simulink model "UUV_PID_Control_Model"  (R2019b)
settings: Solver=VariableStepAuto  StartTime=0.0  StopTime=12  RelTol=1e-3
undefined symbols (not defined in the file): dr, drr, dx, dxx, dz, dzz, g, kdr, kds, kdx, kdz, kf, kir, kis, kix, kiz, kpr, kps, kpx, kpz, L, mr, mx, mz, r, Ud, waypoints
libraries: simulink x2
settings Model: Creator=7385281  LastModifiedBy=7385281
settings SolverCC: ZeroCrossAlgorithm=Adaptive
settings DataIOCC: ReturnWorkspaceOutputs=off
settings DebuggingCC: IgnoredZcDiagnostic=none

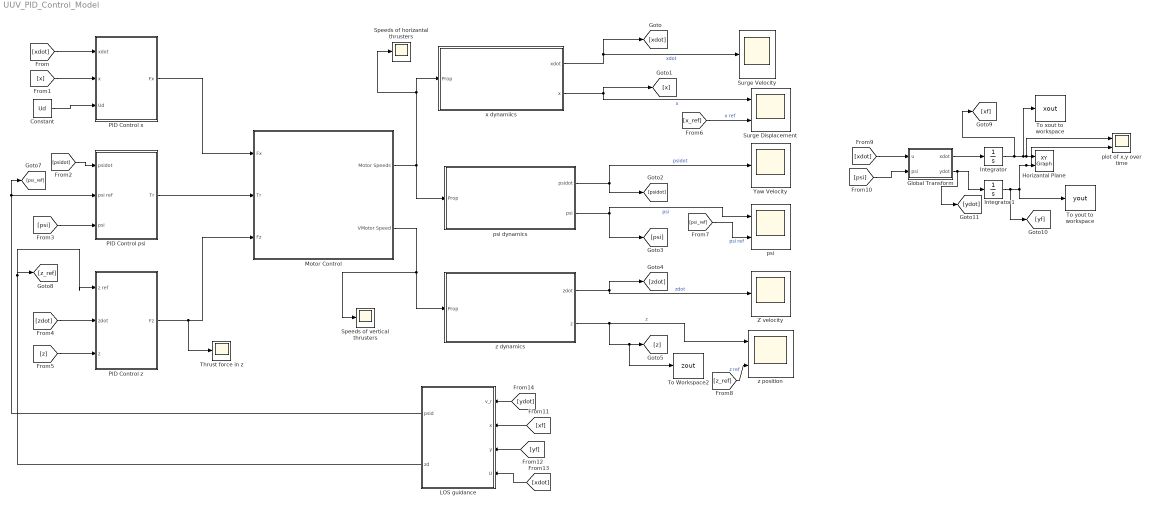
== system UUV_PID_Control_Model ==
  Constant : Constant  Value=Ud
  Global Transform : MATLAB Function  TreatAsAtomicUnit=on
  Horizantal Plane : simulink/Sinks/XY Graph  xmin=-5  xmax=5  ymin=-5  ymax=5  st=-1
  Integrator : Integrator
  Integrator1 : Integrator
  LOS guidance : Subsystem
  Motor Control : Subsystem
  PID Control psi : Subsystem
  PID Control x : Subsystem
  PID Control z : Subsystem
  Speeds of horizantal thrusters : Scope
  Speeds of vertical thrusters : Scope
  Surge Displacement : Scope  NumInputPorts=2
  Surge Velocity : Scope
  Thrust force in z : Scope
  To Workspace2 : ToWorkspace  VariableName=zout  SampleTime=-1
      settings: Save2DSignal=2-D array (concatenate along first dimension)
  To xout to workspace : ToWorkspace  VariableName=xout  SampleTime=-1
      settings: Save2DSignal=2-D array (concatenate along first dimension)
  To yout to workspace : ToWorkspace  VariableName=yout  SampleTime=-1
      settings: Save2DSignal=2-D array (concatenate along first dimension)
  Yaw Velocity : Scope
  Z velocity : Scope
  plot of x,y over time : Scope  NumInputPorts=2
  psi : Scope  NumInputPorts=2
  psi dynamics : Subsystem
  x dynamiics : Subsystem
  z dynamics : Subsystem
  z position : Scope  NumInputPorts=2
  wires:
  x dynamiics/1(xdot) -> [xdot], Surge Velocity/1  "xdot"
  x dynamiics/2(x) -> Surge Displacement/1, [x]  "x"
  psi dynamics/2(psi) -> [psi], psi/1  "psi"
  psi dynamics/1(psidot) -> Yaw Velocity/1, [psidot]  "psidot"
  z dynamics/1(zdot) -> [zdot], Z velocity/1  "zdot"
  z dynamics/2(z) -> z position/1, To Workspace2/1, [z]  "z"
  Motor Control/2(VMotor Speed) -> Speeds of vertical thrusters/1, z dynamics/1(Prop)
  PID Control x/1(Fx) -> Motor Control/1(Fx)
  LOS guidance/1(psid) -> [psi_ref], PID Control psi/2(psi ref)
  PID Control psi/1(Tr) -> Motor Control/2(Tr)
  LOS guidance/2(zd) -> PID Control z/1(z ref), [z_ref]
  PID Control z/1(Fz) -> Thrust force in z/1, Motor Control/3(Fz)
  [xdot] -> PID Control x/1(xdot)
  [x] -> PID Control x/2(x)
  [psidot] -> PID Control psi/1(psidot)
  [psi] -> PID Control psi/3(psi)
  [zdot] -> PID Control z/2(zdot)
  [z] -> PID Control z/3(z)
  [x_ref] -> Surge Displacement/2  "x ref"
  [psi_ref] -> psi/2  "psi ref"
  [z_ref] -> z position/2  "z ref"
  Global Transform/1(xdot) -> Integrator/1
  Global Transform/2(ydot) -> [ydot], Integrator1/1
  [xdot] -> Global Transform/1(u)
  [psi] -> Global Transform/2(psi)
  Integrator/1 -> [xf], To xout to workspace/1, plot of x,y over time/1, Horizantal Plane/1
  Integrator1/1 -> [yf], plot of x,y over time/2, Horizantal Plane/2, To yout to workspace/1
  [xf] -> LOS guidance/2(x)
  [yf] -> LOS guidance/3(y)
  [xdot] -> LOS guidance/4(U)
  [ydot] -> LOS guidance/1(v_r)
  Constant/1 -> PID Control x/3(Ud)
  Motor Control/1(Motor Speeds) -> Speeds of horizantal thrusters/1, x dynamiics/1(Prop), psi dynamics/1(Prop)

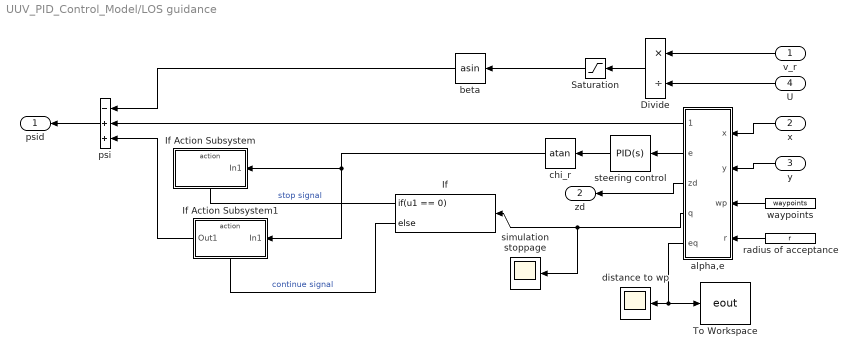
== system UUV_PID_Control_Model/LOS guidance ==
  v_r : Inport
  x : Inport  Port=2
  y : Inport  Port=3
  U : Inport  Port=4
  Divide : Product  Inputs=*/
  If : If  IfExpression=u1 == 0
  If Action Subsystem : Subsystem  TreatAsAtomicUnit=on
  If Action Subsystem1 : Subsystem  TreatAsAtomicUnit=on
  Saturation : Saturate  UpperLimit=1  LowerLimit=-1
  To Workspace : ToWorkspace  VariableName=eout  SampleTime=-1
      settings: Save2DSignal=2-D array (concatenate along first dimension)
  alpha,e : MATLAB Function  TreatAsAtomicUnit=on
  beta : Trigonometry  Operator=asin
  chi_r : Trigonometry  Operator=atan
  distance to wp : Scope
  psi : Sum  Inputs=-++
  radius of acceptance : Constant  Value=r
  simulation stoppage : Scope
  steering control : simulink/Continuous/PID Controller  Controller=PID  Form=Parallel  TimeDomain=Continuous-time  SampleTime=-1  IntegratorMethod=Forward Euler  FilterMethod=Forward Euler  ControllerParametersSource=internal  P=kps  I=kis  D=kds  UseFilter=on  N=100  TunerSelectOption=Transfer Function Based (PID Tuner App)  InitialConditionSource=internal  InitialConditionForIntegrator=0  InitialConditionForFilter=0  DifferentiatorICPrevScaledInput=0  ExternalReset=none  TrackingMode=off  Kt=1  LimitOutput=off  UpperSaturationLimit=inf  LowerSaturationLimit=-inf  LinearizeAsGain=on  AntiWindupMode=none  Kb=1  POutMin=[]  POutMax=[]  IOutMin=[]  IOutMax=[]  DOutMin=[]  DOutMax=[]  NOutMin=[]  NOutMax=[]  SumOutMin=[]  SumOutMax=[]  SaturationOutMin=[]  SaturationOutMax=[]  PParamMin=[]  PParamMax=[]  IParamMin=[]  IParamMax=[]  DParamMin=[]  DParamMax=[]  NParamMin=[]  NParamMax=[]  KbParamMin=[]  KbParamMax=[]  KtParamMin=[]  KtParamMax=[]  KbOutMin=[]  KbOutMax=[]  KtOutMin=[]  KtOutMax=[]  IntegratorOutMin=[]  IntegratorOutMax=[]  FilterOutMin=[]  FilterOutMax=[]  SumI1OutMin=[]  SumI1OutMax=[]  SumI2OutMin=[]  SumI2OutMax=[]  SumI3OutMin=[]  SumI3OutMax=[]  SumI4OutMin=[]  SumI4OutMax=[]  SumDOutMin=[]  SumDOutMax=[]  DifferentiatorOutMin=[]  DifferentiatorOutMax=[]  FilterDiffOutCoefMin=[]  FilterDiffOutCoefMax=[]  ReciprocalOutMin=[]  ReciprocalOutMax=[]  SumDenOutMin=[]  SumDenOutMax=[]  SumNumOutMin=[]  SumNumOutMax=[]  DivideOutMin=[]  DivideOutMax=[]  IntegratorContinuousStateAttributes=''  IntegratorStateMustResolveToSignalObject=off  IntegratorRTWStateStorageClass=Auto  FilterContinuousStateAttributes=''  FilterStateMustResolveToSignalObject=off  FilterRTWStateStorageClass=Auto  ParallelPVariant=InternalParameters  IdealPVariant=Disabled  IVariant=InternalParameters  DVariant=InternalParameters  IntegratorVariant=Continuous  SatVariant=Disabled  AWVariant=Passthrough  PCopyVariant=Disabled  TRVariant=Disabled  FdbkBlocksVariant=Forward  IdealPFdbkVariant=Disabled  SatFdbkVariant=Disabled  DerivativeFilterVariant=ContFilter  NVariant=InternalParameters  NCopyVariant=Disabled  FilterICVariant=InternalICsFilter  IntegratorICVariant=InternalICs  ExternalResetVariant=Disabled  TRSumVariant=Passthrough  SumFdbkVariant=Disabled  SumVariant=Sum_PID
  waypoints : Constant  Value=waypoints
  psid : Outport  VectorParamsAs1DForOutWhenUnconnected=off
  zd : Outport  Port=2  VectorParamsAs1DForOutWhenUnconnected=off
  wires:
  x/1 -> alpha,e/1(x)
  waypoints/1 -> alpha,e/3(wp)
  alpha,e/3(zd) -> zd/1
  alpha,e/2(e) -> steering control/1
  U/1 -> Divide/2
  radius of acceptance/1 -> alpha,e/4(r)
  y/1 -> alpha,e/2(y)
  beta/1 -> psi/1
  v_r/1 -> Divide/1
  Divide/1 -> Saturation/1
  steering control/1 -> chi_r/1
  alpha,e/1(alpha) -> psi/2
  chi_r/1 -> If Action Subsystem1/1(In1), If Action Subsystem/1(In1)
  psi/1 -> psid/1
  Saturation/1 -> beta/1
  alpha,e/4(q) -> If/1, simulation stoppage/1
  If/1 -> If Action Subsystem/Action  "stop signal"
  If/2 -> If Action Subsystem1/Action  "continue signal"
  If Action Subsystem1/1(Out1) -> psi/3
  alpha,e/5(eq) -> To Workspace/1, distance to wp/1

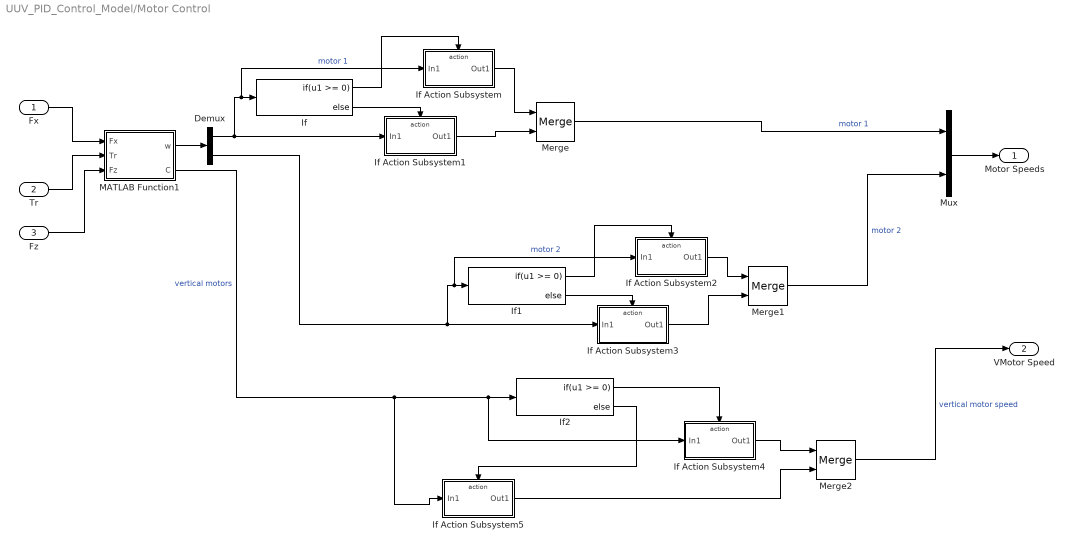
== system UUV_PID_Control_Model/Motor Control ==
  Fx : Inport
  Tr : Inport  Port=2
  Fz : Inport  Port=3
  Demux : Demux  Outputs=2
  If : If  IfExpression=u1 >= 0
  If Action Subsystem : Subsystem  TreatAsAtomicUnit=on
  If Action Subsystem1 : Subsystem  TreatAsAtomicUnit=on
  If Action Subsystem2 : Subsystem  TreatAsAtomicUnit=on
  If Action Subsystem3 : Subsystem  TreatAsAtomicUnit=on
  If Action Subsystem4 : Subsystem  TreatAsAtomicUnit=on
  If Action Subsystem5 : Subsystem  TreatAsAtomicUnit=on
  If1 : If  IfExpression=u1 >= 0
  If2 : If  IfExpression=u1 >= 0
  MATLAB Function1 : MATLAB Function  TreatAsAtomicUnit=on
  Merge : Merge
  Merge1 : Merge
  Merge2 : Merge
  Mux : Mux  Inputs=2
  Motor Speeds : Outport
  VMotor Speed : Outport  Port=2
  wires:
  If Action Subsystem1/1(Out1) -> Merge/2
  If Action Subsystem/1(Out1) -> Merge/1
  If1/1 -> If Action Subsystem2/Action
  If Action Subsystem3/1(Out1) -> Merge1/2
  If/2 -> If Action Subsystem1/Action
  MATLAB Function1/1(w) -> Demux/1
  Demux/1 -> If Action Subsystem/1(In1), If/1, If Action Subsystem1/1(In1)  "motor 1"
  If1/2 -> If Action Subsystem3/Action
  If Action Subsystem2/1(Out1) -> Merge1/1
  Merge1/1 -> Mux/2  "motor 2"
  If/1 -> If Action Subsystem/Action
  Demux/2 -> If Action Subsystem2/1(In1), If1/1, If Action Subsystem3/1(In1)  "motor 2"
  Merge/1 -> Mux/1  "motor 1"
  Tr/1 -> MATLAB Function1/2(Tr)
  Fx/1 -> MATLAB Function1/1(Fx)
  Mux/1 -> Motor Speeds/1
  Fz/1 -> MATLAB Function1/3(Fz)
  Merge2/1 -> VMotor Speed/1  "vertical motor speed"
  MATLAB Function1/2(C) -> If Action Subsystem5/1(In1), If Action Subsystem4/1(In1), If2/1  "vertical motors"
  If Action Subsystem4/1(Out1) -> Merge2/1
  If2/2 -> If Action Subsystem5/Action
  If2/1 -> If Action Subsystem4/Action
  If Action Subsystem5/1(Out1) -> Merge2/2

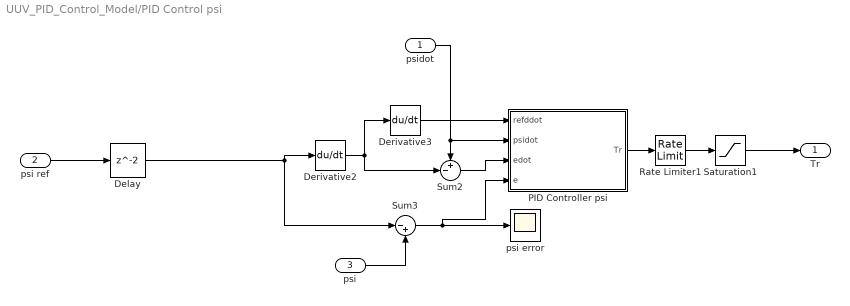
== system UUV_PID_Control_Model/PID Control psi ==
  psidot : Inport
  psi ref : Inport  Port=2
  psi : Inport  Port=3
  Delay : Delay
  Derivative2 : Derivative
  Derivative3 : Derivative
  PID Controller psi : Subsystem
  Rate Limiter1 : RateLimiter  RisingSlewLimit=100  FallingSlewLimit=-100  SampleTimeMode=inherited
  Saturation1 : Saturate  UpperLimit=100  LowerLimit=-100
  Sum2 : Sum  Inputs=+-|
  Sum3 : Sum  Inputs=|-+
  psi error : Scope
  Tr : Outport
  wires:
  PID Controller psi/1(Tr) -> Rate Limiter1/1
  Derivative2/1 -> Sum2/2, Derivative3/1
  Sum3/1 -> PID Controller psi/4(e), psi error/1
  Derivative3/1 -> PID Controller psi/1(refddot)
  psi ref/1 -> Delay/1
  psi/1 -> Sum3/2
  Sum2/1 -> PID Controller psi/3(edot)
  psidot/1 -> Sum2/1, PID Controller psi/2(psidot)
  Rate Limiter1/1 -> Saturation1/1
  Saturation1/1 -> Tr/1
  Delay/1 -> Derivative2/1, Sum3/1

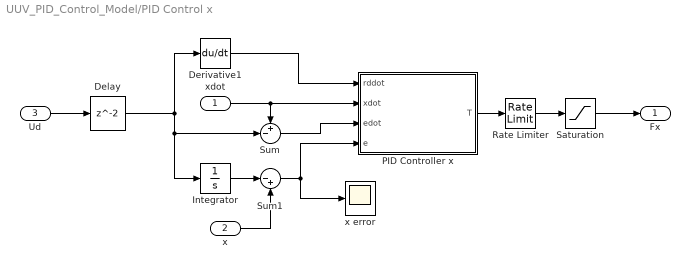
== system UUV_PID_Control_Model/PID Control x ==
  xdot : Inport
  x : Inport  Port=2
  Ud : Inport  Port=3
  Delay : Delay
  Derivative1 : Derivative
  Integrator : Integrator
  PID Controller x : Subsystem
  Rate Limiter : RateLimiter  RisingSlewLimit=100  FallingSlewLimit=-100  SampleTimeMode=inherited
  Saturation : Saturate  UpperLimit=100  LowerLimit=-100
  Sum : Sum  Inputs=+-|
  Sum1 : Sum  Inputs=|-+
  x error : Scope
  Fx : Outport
  wires:
  Sum1/1 -> PID Controller x/4(e), x error/1
  PID Controller x/1(T) -> Rate Limiter/1
  Sum/1 -> PID Controller x/3(edot)
  Ud/1 -> Delay/1
  Rate Limiter/1 -> Saturation/1
  Saturation/1 -> Fx/1
  xdot/1 -> Sum/1, PID Controller x/2(xdot)
  Derivative1/1 -> PID Controller x/1(rddot)
  x/1 -> Sum1/2
  Integrator/1 -> Sum1/1
  Delay/1 -> Integrator/1, Sum/2, Derivative1/1

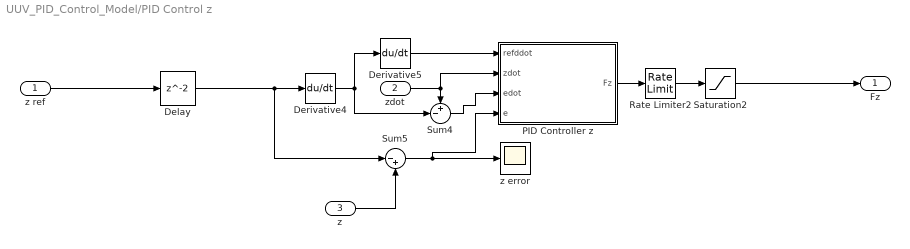
== system UUV_PID_Control_Model/PID Control z ==
  z ref : Inport
  zdot : Inport  Port=2
  z : Inport  Port=3
  Delay : Delay
  Derivative4 : Derivative
  Derivative5 : Derivative
  PID Controller z : Subsystem
  Rate Limiter2 : RateLimiter  RisingSlewLimit=100  FallingSlewLimit=-100  SampleTimeMode=inherited
  Saturation2 : Saturate  UpperLimit=100  LowerLimit=-100
  Sum4 : Sum  Inputs=+-|
  Sum5 : Sum  Inputs=|-+
  z error : Scope
  Fz : Outport
  wires:
  PID Controller z/1(Fz) -> Rate Limiter2/1
  Sum5/1 -> PID Controller z/4(e), z error/1
  zdot/1 -> PID Controller z/2(zdot), Sum4/1
  Derivative4/1 -> Sum4/2, Derivative5/1
  Derivative5/1 -> PID Controller z/1(refddot)
  Rate Limiter2/1 -> Saturation2/1
  z ref/1 -> Delay/1
  Sum4/1 -> PID Controller z/3(edot)
  z/1 -> Sum5/2
  Saturation2/1 -> Fz/1
  Delay/1 -> Sum5/1, Derivative4/1

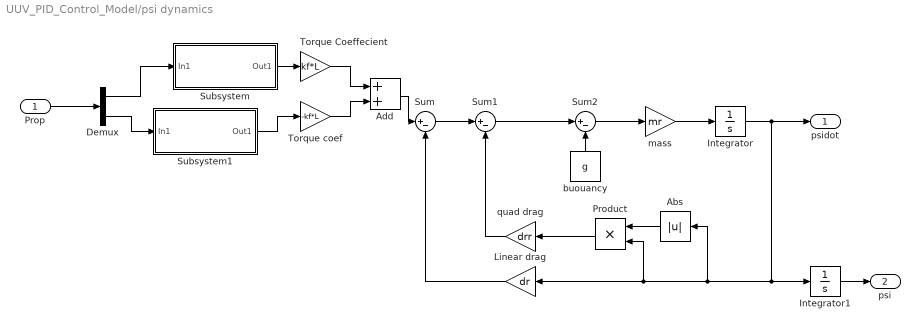
== system UUV_PID_Control_Model/psi dynamics ==
  Prop : Inport
  Abs : Abs
  Add : Sum
  Demux : Demux  Outputs=2
  Integrator : Integrator
  Integrator1 : Integrator
  Linear drag : Gain  Gain=dr
  Product : Product
  Subsystem : Subsystem
  Subsystem1 : Subsystem
  Sum : Sum  Inputs=|+-
  Sum1 : Sum  Inputs=|+-
  Sum2 : Sum  Inputs=|+-
  Torque Coeffecient : Gain  Gain=kf*L
  Torque coef : Gain  Gain=-kf*L
  buouancy : Constant  Value=g
  mass : Gain  Gain=mr
  quad drag : Gain  Gain=drr
  psidot : Outport
  psi : Outport  Port=2
  wires:
  Sum1/1 -> Sum2/1
  Sum/1 -> Sum1/1
  buouancy/1 -> Sum2/2
  Sum2/1 -> mass/1
  mass/1 -> Integrator/1
  Integrator/1 -> Abs/1, Product/2, Linear drag/1, Integrator1/1, psidot/1
  Abs/1 -> Product/1
  Product/1 -> quad drag/1
  quad drag/1 -> Sum1/2
  Linear drag/1 -> Sum/2
  Integrator1/1 -> psi/1
  Prop/1 -> Demux/1
  Demux/1 -> Subsystem/1(In1)
  Demux/2 -> Subsystem1/1(In1)
  Subsystem/1(Out1) -> Torque Coeffecient/1
  Subsystem1/1(Out1) -> Torque coef/1
  Torque Coeffecient/1 -> Add/1
  Torque coef/1 -> Add/2
  Add/1 -> Sum/1

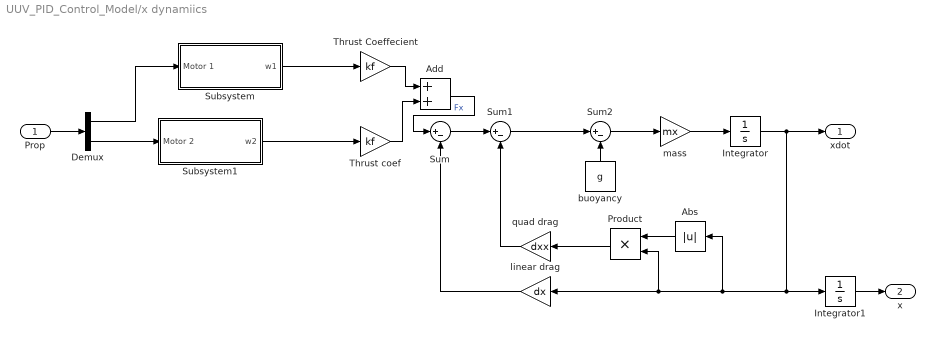
== system UUV_PID_Control_Model/x dynamiics ==
  Prop : Inport
  Abs : Abs
  Add : Sum
  Demux : Demux  Outputs=2
  Integrator : Integrator  InitialCondition=0.001
  Integrator1 : Integrator
  Product : Product
  Subsystem : Subsystem
  Subsystem1 : Subsystem
  Sum : Sum  Inputs=|+-
  Sum1 : Sum  Inputs=|+-
  Sum2 : Sum  Inputs=|+-
  Thrust Coeffecient : Gain  Gain=kf
  Thrust coef : Gain  Gain=kf
  buoyancy : Constant  Value=g
  linear drag : Gain  Gain=dx
  mass : Gain  Gain=mx
  quad drag : Gain  Gain=dxx
  xdot : Outport
  x : Outport  Port=2
  wires:
  Sum1/1 -> Sum2/1
  Sum/1 -> Sum1/1
  buoyancy/1 -> Sum2/2
  Sum2/1 -> mass/1
  mass/1 -> Integrator/1
  Integrator/1 -> Abs/1, Product/2, linear drag/1, Integrator1/1, xdot/1
  Abs/1 -> Product/1
  Product/1 -> quad drag/1
  quad drag/1 -> Sum1/2
  linear drag/1 -> Sum/2
  Integrator1/1 -> x/1
  Prop/1 -> Demux/1
  Subsystem/1(w1) -> Thrust Coeffecient/1
  Demux/2 -> Subsystem1/1(Motor 2)
  Subsystem1/1(w2) -> Thrust coef/1
  Thrust Coeffecient/1 -> Add/1
  Thrust coef/1 -> Add/2
  Add/1 -> Sum/1  "Fx"
  Demux/1 -> Subsystem/1(Motor 1)

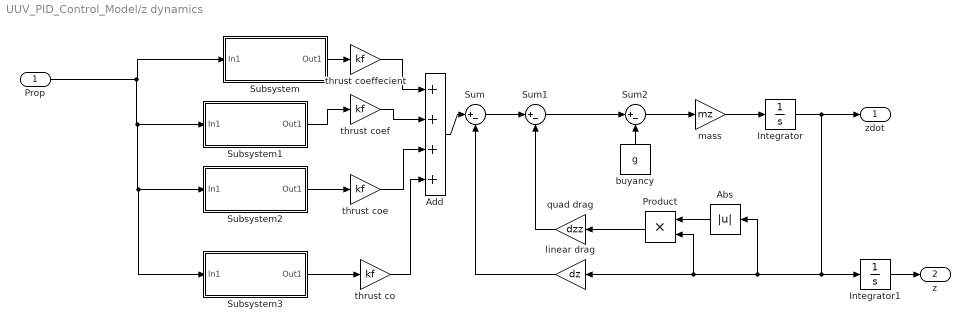
== system UUV_PID_Control_Model/z dynamics ==
  Prop : Inport
  Abs : Abs
  Add : Sum  Inputs=++++
  Integrator : Integrator
  Integrator1 : Integrator
  Product : Product
  Subsystem : Subsystem
  Subsystem1 : Subsystem
  Subsystem2 : Subsystem
  Subsystem3 : Subsystem
  Sum : Sum  Inputs=|+-
  Sum1 : Sum  Inputs=|+-
  Sum2 : Sum  Inputs=|+-
  buyancy : Constant  Value=g
  linear drag : Gain  Gain=dz
  mass : Gain  Gain=mz
  quad drag : Gain  Gain=dzz
  thrust co : Gain  Gain=kf
  thrust coe : Gain  Gain=kf
  thrust coef : Gain  Gain=kf
  thrust coeffecient : Gain  Gain=kf
  zdot : Outport
  z : Outport  Port=2
  wires:
  Sum1/1 -> Sum2/1
  Sum/1 -> Sum1/1
  buyancy/1 -> Sum2/2
  Sum2/1 -> mass/1
  mass/1 -> Integrator/1
  Integrator/1 -> Abs/1, Product/2, linear drag/1, Integrator1/1, zdot/1
  Abs/1 -> Product/1
  Product/1 -> quad drag/1
  quad drag/1 -> Sum1/2
  linear drag/1 -> Sum/2
  Integrator1/1 -> z/1
  Subsystem/1(Out1) -> thrust coeffecient/1
  Subsystem1/1(Out1) -> thrust coef/1
  thrust coeffecient/1 -> Add/1
  thrust coef/1 -> Add/2
  Add/1 -> Sum/1
  Subsystem2/1(Out1) -> thrust coe/1
  thrust coe/1 -> Add/3
  thrust co/1 -> Add/4
  Subsystem3/1(Out1) -> thrust co/1
  Prop/1 -> Subsystem3/1(In1), Subsystem2/1(In1), Subsystem1/1(In1), Subsystem/1(In1)

== system UUV_PID_Control_Model/LOS guidance/If Action Subsystem ==
  In1 : Inport
  Action Port : ActionPort  ActionPortLabel=if(u1 == 0)
  Stop Simulation : Stop
  wires:
  In1/1 -> Stop Simulation/1

== system UUV_PID_Control_Model/LOS guidance/If Action Subsystem1 ==
  In1 : Inport
  Action Port : ActionPort  ActionPortLabel=else
  Out1 : Outport
  wires:
  In1/1 -> Out1/1

== system UUV_PID_Control_Model/Motor Control/If Action Subsystem ==
  In1 : Inport
  Action Port : ActionPort  ActionPortLabel=if(u1 >= 0)
  Square Root : Sqrt  SaturateOnIntegerOverflow=on
  Out1 : Outport
  wires:
  In1/1 -> Square Root/1
  Square Root/1 -> Out1/1

== system UUV_PID_Control_Model/Motor Control/If Action Subsystem1 ==
  In1 : Inport
  Action Port : ActionPort  ActionPortLabel=else
  Abs : Abs
  Gain : Gain  Gain=-1
  Square Root : Sqrt  SaturateOnIntegerOverflow=on
  Out1 : Outport
  wires:
  In1/1 -> Abs/1
  Abs/1 -> Square Root/1
  Square Root/1 -> Gain/1
  Gain/1 -> Out1/1

== system UUV_PID_Control_Model/Motor Control/If Action Subsystem2 ==
  In1 : Inport
  Action Port : ActionPort  ActionPortLabel=if(u1 >= 0)
  Square Root : Sqrt  SaturateOnIntegerOverflow=on
  Out1 : Outport
  wires:
  In1/1 -> Square Root/1
  Square Root/1 -> Out1/1

== system UUV_PID_Control_Model/Motor Control/If Action Subsystem3 ==
  In1 : Inport
  Action Port : ActionPort  ActionPortLabel=else
  Abs : Abs
  Gain : Gain  Gain=-1
  Square Root : Sqrt  SaturateOnIntegerOverflow=on
  Out1 : Outport
  wires:
  In1/1 -> Abs/1
  Abs/1 -> Square Root/1
  Square Root/1 -> Gain/1
  Gain/1 -> Out1/1

== system UUV_PID_Control_Model/Motor Control/If Action Subsystem4 ==
  In1 : Inport
  Action Port : ActionPort  ActionPortLabel=if(u1 >= 0)
  Square Root : Sqrt  SaturateOnIntegerOverflow=on
  Out1 : Outport
  wires:
  In1/1 -> Square Root/1
  Square Root/1 -> Out1/1

== system UUV_PID_Control_Model/Motor Control/If Action Subsystem5 ==
  In1 : Inport
  Action Port : ActionPort  ActionPortLabel=else
  Abs : Abs
  Gain : Gain  Gain=-1
  Square Root : Sqrt  SaturateOnIntegerOverflow=on
  Out1 : Outport
  wires:
  In1/1 -> Abs/1
  Abs/1 -> Square Root/1
  Square Root/1 -> Gain/1
  Gain/1 -> Out1/1

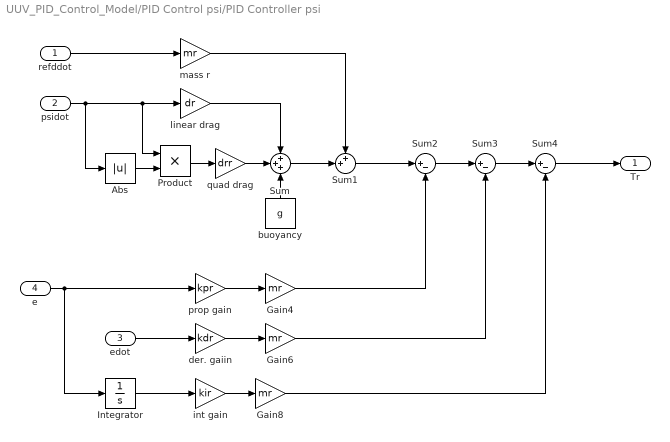
== system UUV_PID_Control_Model/PID Control psi/PID Controller psi ==
  refddot : Inport
  psidot : Inport  Port=2
  edot : Inport  Port=3
  e : Inport  Port=4
  Abs : Abs
  Gain4 : Gain  Gain=mr
  Gain6 : Gain  Gain=mr
  Gain8 : Gain  Gain=mr
  Integrator : Integrator
  Product : Product
  Sum : Sum  Inputs=+++
  Sum1 : Sum  Inputs=++|
  Sum2 : Sum  Inputs=|+-
  Sum3 : Sum  Inputs=|+-
  Sum4 : Sum  Inputs=|+-
  buoyancy : Constant  Value=g
  der. gaiin : Gain  Gain=kdr
  int gain : Gain  Gain=kir
  linear drag : Gain  Gain=dr
  mass r : Gain  Gain=mr
  prop gain : Gain  Gain=kpr
  quad drag : Gain  Gain=drr
  Tr : Outport
  wires:
  psidot/1 -> Product/1, linear drag/1, Abs/1
  Abs/1 -> Product/2
  refddot/1 -> mass r/1
  Product/1 -> quad drag/1
  quad drag/1 -> Sum/2
  linear drag/1 -> Sum/1
  buoyancy/1 -> Sum/3
  Sum/1 -> Sum1/2
  mass r/1 -> Sum1/1
  Sum1/1 -> Sum2/1
  e/1 -> Integrator/1, prop gain/1
  prop gain/1 -> Gain4/1
  Gain4/1 -> Sum2/2
  edot/1 -> der. gaiin/1
  der. gaiin/1 -> Gain6/1
  Integrator/1 -> int gain/1
  int gain/1 -> Gain8/1
  Sum2/1 -> Sum3/1
  Gain6/1 -> Sum3/2
  Gain8/1 -> Sum4/2
  Sum3/1 -> Sum4/1
  Sum4/1 -> Tr/1

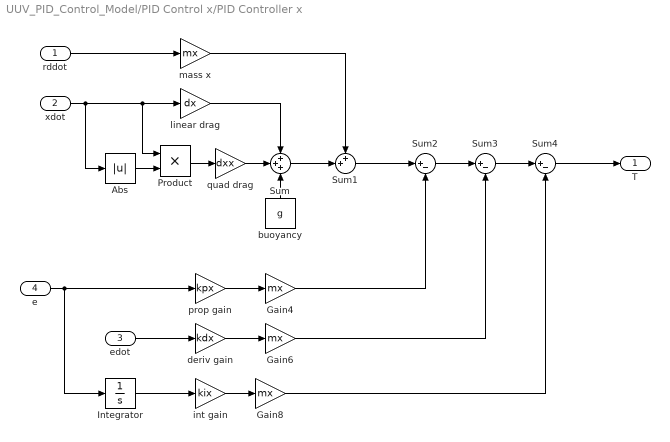
== system UUV_PID_Control_Model/PID Control x/PID Controller x ==
  rddot : Inport
  xdot : Inport  Port=2
  edot : Inport  Port=3
  e : Inport  Port=4
  Abs : Abs
  Gain4 : Gain  Gain=mx
  Gain6 : Gain  Gain=mx
  Gain8 : Gain  Gain=mx
  Integrator : Integrator
  Product : Product
  Sum : Sum  Inputs=+++
  Sum1 : Sum  Inputs=++|
  Sum2 : Sum  Inputs=|+-
  Sum3 : Sum  Inputs=|+-
  Sum4 : Sum  Inputs=|+-
  buoyancy : Constant  Value=g
  deriv gain : Gain  Gain=kdx
  int gain : Gain  Gain=kix
  linear drag : Gain  Gain=dx
  mass x : Gain  Gain=mx
  prop gain : Gain  Gain=kpx
  quad drag : Gain  Gain=dxx
  T : Outport
  wires:
  xdot/1 -> Product/1, linear drag/1, Abs/1
  Abs/1 -> Product/2
  rddot/1 -> mass x/1
  Product/1 -> quad drag/1
  quad drag/1 -> Sum/2
  linear drag/1 -> Sum/1
  buoyancy/1 -> Sum/3
  Sum/1 -> Sum1/2
  mass x/1 -> Sum1/1
  Sum1/1 -> Sum2/1
  e/1 -> Integrator/1, prop gain/1
  prop gain/1 -> Gain4/1
  Gain4/1 -> Sum2/2
  edot/1 -> deriv gain/1
  deriv gain/1 -> Gain6/1
  Integrator/1 -> int gain/1
  int gain/1 -> Gain8/1
  Sum2/1 -> Sum3/1
  Gain6/1 -> Sum3/2
  Gain8/1 -> Sum4/2
  Sum3/1 -> Sum4/1
  Sum4/1 -> T/1

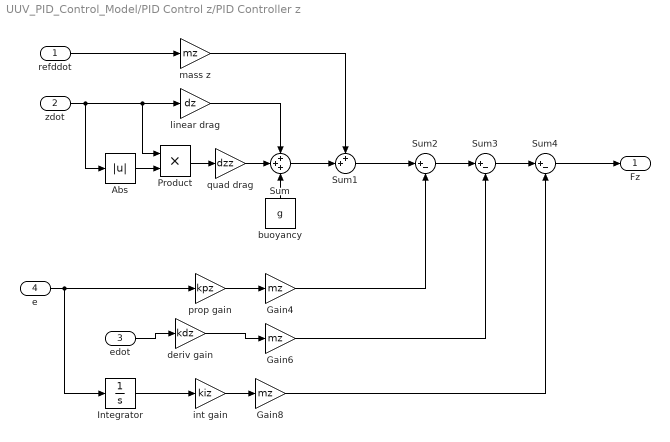
== system UUV_PID_Control_Model/PID Control z/PID Controller z ==
  refddot : Inport
  zdot : Inport  Port=2
  edot : Inport  Port=3
  e : Inport  Port=4
  Abs : Abs
  Gain4 : Gain  Gain=mz
  Gain6 : Gain  Gain=mz
  Gain8 : Gain  Gain=mz
  Integrator : Integrator
  Product : Product
  Sum : Sum  Inputs=+++
  Sum1 : Sum  Inputs=++|
  Sum2 : Sum  Inputs=|+-
  Sum3 : Sum  Inputs=|+-
  Sum4 : Sum  Inputs=|+-
  buoyancy : Constant  Value=g
  deriv gain : Gain  Gain=kdz
  int gain : Gain  Gain=kiz
  linear drag : Gain  Gain=dz
  mass z : Gain  Gain=mz
  prop gain : Gain  Gain=kpz
  quad drag : Gain  Gain=dzz
  Fz : Outport
  wires:
  zdot/1 -> Product/1, linear drag/1, Abs/1
  Abs/1 -> Product/2
  refddot/1 -> mass z/1
  Product/1 -> quad drag/1
  quad drag/1 -> Sum/2
  linear drag/1 -> Sum/1
  buoyancy/1 -> Sum/3
  Sum/1 -> Sum1/2
  mass z/1 -> Sum1/1
  Sum1/1 -> Sum2/1
  e/1 -> Integrator/1, prop gain/1
  prop gain/1 -> Gain4/1
  Gain4/1 -> Sum2/2
  edot/1 -> deriv gain/1
  deriv gain/1 -> Gain6/1
  Integrator/1 -> int gain/1
  int gain/1 -> Gain8/1
  Sum2/1 -> Sum3/1
  Gain6/1 -> Sum3/2
  Gain8/1 -> Sum4/2
  Sum3/1 -> Sum4/1
  Sum4/1 -> Fz/1

== system UUV_PID_Control_Model/psi dynamics/Subsystem ==
  In1 : Inport
  If : If  IfExpression=u1 >= 0
  If Action Subsystem : Subsystem  TreatAsAtomicUnit=on
  If Action Subsystem1 : Subsystem  TreatAsAtomicUnit=on
  Merge : Merge
  Out1 : Outport
  wires:
  In1/1 -> If Action Subsystem1/1(In1), If Action Subsystem/1(In1), If/1
  If/1 -> If Action Subsystem/Action
  If/2 -> If Action Subsystem1/Action
  If Action Subsystem/1(Out1) -> Merge/1
  If Action Subsystem1/1(Out1) -> Merge/2
  Merge/1 -> Out1/1

== system UUV_PID_Control_Model/psi dynamics/Subsystem1 ==
  In1 : Inport
  If : If  IfExpression=u1 >= 0
  If Action Subsystem : Subsystem  TreatAsAtomicUnit=on
  If Action Subsystem1 : Subsystem  TreatAsAtomicUnit=on
  Merge : Merge
  Out1 : Outport
  wires:
  In1/1 -> If Action Subsystem1/1(In1), If Action Subsystem/1(In1), If/1
  If/1 -> If Action Subsystem/Action
  If/2 -> If Action Subsystem1/Action
  If Action Subsystem/1(Out1) -> Merge/1
  If Action Subsystem1/1(Out1) -> Merge/2
  Merge/1 -> Out1/1

== system UUV_PID_Control_Model/x dynamiics/Subsystem ==
  Motor 1 : Inport
  If : If  IfExpression=u1 >= 0
  If Action Subsystem : Subsystem  TreatAsAtomicUnit=on
  If Action Subsystem1 : Subsystem  TreatAsAtomicUnit=on
  Merge : Merge
  w1 : Outport
  wires:
  Motor 1/1 -> If Action Subsystem1/1(In1), If Action Subsystem/1(In1), If/1
  If/1 -> If Action Subsystem/Action
  If/2 -> If Action Subsystem1/Action
  If Action Subsystem/1(Out1) -> Merge/1
  If Action Subsystem1/1(Out1) -> Merge/2
  Merge/1 -> w1/1  "w1"

== system UUV_PID_Control_Model/x dynamiics/Subsystem1 ==
  Motor 2 : Inport
  If : If  IfExpression=u1 >= 0
  If Action Subsystem : Subsystem  TreatAsAtomicUnit=on
  If Action Subsystem1 : Subsystem  TreatAsAtomicUnit=on
  Merge : Merge
  w2 : Outport
  wires:
  Motor 2/1 -> If Action Subsystem1/1(In1), If Action Subsystem/1(In1), If/1
  If/1 -> If Action Subsystem/Action
  If/2 -> If Action Subsystem1/Action
  If Action Subsystem/1(Out1) -> Merge/1
  If Action Subsystem1/1(Out1) -> Merge/2
  Merge/1 -> w2/1  "w2"

== system UUV_PID_Control_Model/z dynamics/Subsystem ==
  In1 : Inport
  If : If  IfExpression=u1 >= 0
  If Action Subsystem : Subsystem  TreatAsAtomicUnit=on
  If Action Subsystem1 : Subsystem  TreatAsAtomicUnit=on
  Merge : Merge
  Out1 : Outport
  wires:
  In1/1 -> If Action Subsystem1/1(In1), If Action Subsystem/1(In1), If/1
  If/1 -> If Action Subsystem/Action
  If/2 -> If Action Subsystem1/Action
  If Action Subsystem/1(Out1) -> Merge/1
  If Action Subsystem1/1(Out1) -> Merge/2
  Merge/1 -> Out1/1

== system UUV_PID_Control_Model/z dynamics/Subsystem1 ==
  In1 : Inport
  If : If  IfExpression=u1 >= 0
  If Action Subsystem : Subsystem  TreatAsAtomicUnit=on
  If Action Subsystem1 : Subsystem  TreatAsAtomicUnit=on
  Merge : Merge
  Out1 : Outport
  wires:
  In1/1 -> If Action Subsystem1/1(In1), If Action Subsystem/1(In1), If/1
  If/1 -> If Action Subsystem/Action
  If/2 -> If Action Subsystem1/Action
  If Action Subsystem/1(Out1) -> Merge/1
  If Action Subsystem1/1(Out1) -> Merge/2
  Merge/1 -> Out1/1

== system UUV_PID_Control_Model/z dynamics/Subsystem2 ==
  In1 : Inport
  If : If  IfExpression=u1 >= 0
  If Action Subsystem : Subsystem  TreatAsAtomicUnit=on
  If Action Subsystem1 : Subsystem  TreatAsAtomicUnit=on
  Merge : Merge
  Out1 : Outport
  wires:
  In1/1 -> If Action Subsystem1/1(In1), If Action Subsystem/1(In1), If/1
  If/1 -> If Action Subsystem/Action
  If/2 -> If Action Subsystem1/Action
  If Action Subsystem/1(Out1) -> Merge/1
  If Action Subsystem1/1(Out1) -> Merge/2
  Merge/1 -> Out1/1

== system UUV_PID_Control_Model/z dynamics/Subsystem3 ==
  In1 : Inport
  If : If  IfExpression=u1 >= 0
  If Action Subsystem : Subsystem  TreatAsAtomicUnit=on
  If Action Subsystem1 : Subsystem  TreatAsAtomicUnit=on
  Merge : Merge
  Out1 : Outport
  wires:
  In1/1 -> If Action Subsystem1/1(In1), If Action Subsystem/1(In1), If/1
  If/1 -> If Action Subsystem/Action
  If/2 -> If Action Subsystem1/Action
  If Action Subsystem/1(Out1) -> Merge/1
  If Action Subsystem1/1(Out1) -> Merge/2
  Merge/1 -> Out1/1

== system UUV_PID_Control_Model/psi dynamics/Subsystem/If Action Subsystem ==
  In1 : Inport
  Action Port : ActionPort  ActionPortLabel=if(u1 >= 0)
  Square : Math  Operator=square  SignedPower=off  SaturateOnIntegerOverflow=on
  Out1 : Outport
  wires:
  In1/1 -> Square/1
  Square/1 -> Out1/1

== system UUV_PID_Control_Model/psi dynamics/Subsystem/If Action Subsystem1 ==
  In1 : Inport
  Action Port : ActionPort  ActionPortLabel=else
  Gain : Gain  Gain=-1
  Square : Math  Operator=square  SignedPower=off  SaturateOnIntegerOverflow=on
  Out1 : Outport
  wires:
  In1/1 -> Square/1
  Gain/1 -> Out1/1
  Square/1 -> Gain/1

== system UUV_PID_Control_Model/psi dynamics/Subsystem1/If Action Subsystem ==
  In1 : Inport
  Action Port : ActionPort  ActionPortLabel=if(u1 >= 0)
  Square : Math  Operator=square  SignedPower=off  SaturateOnIntegerOverflow=on
  Out1 : Outport
  wires:
  In1/1 -> Square/1
  Square/1 -> Out1/1

== system UUV_PID_Control_Model/psi dynamics/Subsystem1/If Action Subsystem1 ==
  In1 : Inport
  Action Port : ActionPort  ActionPortLabel=else
  Gain : Gain  Gain=-1
  Square : Math  Operator=square  SignedPower=off  SaturateOnIntegerOverflow=on
  Out1 : Outport
  wires:
  In1/1 -> Square/1
  Gain/1 -> Out1/1
  Square/1 -> Gain/1

== system UUV_PID_Control_Model/x dynamiics/Subsystem/If Action Subsystem ==
  In1 : Inport
  Action Port : ActionPort  ActionPortLabel=if(u1 >= 0)
  Square : Math  Operator=square  SignedPower=off  SaturateOnIntegerOverflow=on
  Out1 : Outport
  wires:
  In1/1 -> Square/1
  Square/1 -> Out1/1

== system UUV_PID_Control_Model/x dynamiics/Subsystem/If Action Subsystem1 ==
  In1 : Inport
  Action Port : ActionPort  ActionPortLabel=else
  Gain : Gain  Gain=-1
  Square : Math  Operator=square  SignedPower=off  SaturateOnIntegerOverflow=on
  Out1 : Outport
  wires:
  In1/1 -> Square/1
  Gain/1 -> Out1/1
  Square/1 -> Gain/1

== system UUV_PID_Control_Model/x dynamiics/Subsystem1/If Action Subsystem ==
  In1 : Inport
  Action Port : ActionPort  ActionPortLabel=if(u1 >= 0)
  Square : Math  Operator=square  SignedPower=off  SaturateOnIntegerOverflow=on
  Out1 : Outport
  wires:
  In1/1 -> Square/1
  Square/1 -> Out1/1

== system UUV_PID_Control_Model/x dynamiics/Subsystem1/If Action Subsystem1 ==
  In1 : Inport
  Action Port : ActionPort  ActionPortLabel=else
  Gain : Gain  Gain=-1
  Square : Math  Operator=square  SignedPower=off  SaturateOnIntegerOverflow=on
  Out1 : Outport
  wires:
  In1/1 -> Square/1
  Gain/1 -> Out1/1
  Square/1 -> Gain/1

== system UUV_PID_Control_Model/z dynamics/Subsystem/If Action Subsystem ==
  In1 : Inport
  Action Port : ActionPort  ActionPortLabel=if(u1 >= 0)
  Square : Math  Operator=square  SignedPower=off  SaturateOnIntegerOverflow=on
  Out1 : Outport
  wires:
  In1/1 -> Square/1
  Square/1 -> Out1/1

== system UUV_PID_Control_Model/z dynamics/Subsystem/If Action Subsystem1 ==
  In1 : Inport
  Action Port : ActionPort  ActionPortLabel=else
  Gain : Gain  Gain=-1
  Square : Math  Operator=square  SignedPower=off  SaturateOnIntegerOverflow=on
  Out1 : Outport
  wires:
  In1/1 -> Square/1
  Gain/1 -> Out1/1
  Square/1 -> Gain/1

== system UUV_PID_Control_Model/z dynamics/Subsystem1/If Action Subsystem ==
  In1 : Inport
  Action Port : ActionPort  ActionPortLabel=if(u1 >= 0)
  Square : Math  Operator=square  SignedPower=off  SaturateOnIntegerOverflow=on
  Out1 : Outport
  wires:
  In1/1 -> Square/1
  Square/1 -> Out1/1

== system UUV_PID_Control_Model/z dynamics/Subsystem1/If Action Subsystem1 ==
  In1 : Inport
  Action Port : ActionPort  ActionPortLabel=else
  Gain : Gain  Gain=-1
  Square : Math  Operator=square  SignedPower=off  SaturateOnIntegerOverflow=on
  Out1 : Outport
  wires:
  In1/1 -> Square/1
  Gain/1 -> Out1/1
  Square/1 -> Gain/1

== system UUV_PID_Control_Model/z dynamics/Subsystem2/If Action Subsystem ==
  In1 : Inport
  Action Port : ActionPort  ActionPortLabel=if(u1 >= 0)
  Square : Math  Operator=square  SignedPower=off  SaturateOnIntegerOverflow=on
  Out1 : Outport
  wires:
  In1/1 -> Square/1
  Square/1 -> Out1/1

== system UUV_PID_Control_Model/z dynamics/Subsystem2/If Action Subsystem1 ==
  In1 : Inport
  Action Port : ActionPort  ActionPortLabel=else
  Gain : Gain  Gain=-1
  Square : Math  Operator=square  SignedPower=off  SaturateOnIntegerOverflow=on
  Out1 : Outport
  wires:
  In1/1 -> Square/1
  Gain/1 -> Out1/1
  Square/1 -> Gain/1

== system UUV_PID_Control_Model/z dynamics/Subsystem3/If Action Subsystem ==
  In1 : Inport
  Action Port : ActionPort  ActionPortLabel=if(u1 >= 0)
  Square : Math  Operator=square  SignedPower=off  SaturateOnIntegerOverflow=on
  Out1 : Outport
  wires:
  In1/1 -> Square/1
  Square/1 -> Out1/1

== system UUV_PID_Control_Model/z dynamics/Subsystem3/If Action Subsystem1 ==
  In1 : Inport
  Action Port : ActionPort  ActionPortLabel=else
  Gain : Gain  Gain=-1
  Square : Math  Operator=square  SignedPower=off  SaturateOnIntegerOverflow=on
  Out1 : Outport
  wires:
  In1/1 -> Square/1
  Gain/1 -> Out1/1
  Square/1 -> Gain/1

== matlab function UUV_PID_Control_Model/Motor Control/MATLAB Function1 ==
  data: Fx input; w output; Tr input; Fz input; C output
function [w,C] = fcn(Fx,Tr,Fz)
%%%%%%%%%%%%%%%%%%%
% This function takes in the desired forces and torques and maps the forces
% to the 6 proppellers on the hovering UUV, outputting the squared angular
% velocities
%%%%%%%%%%%%%%%%%%%
% Inputs: 
% Fx - desired force in surge
% Tr - desired torque about z 
% Fz - desired force in z
%%%%%%%%%%%%%%%%%%%
% Outputs:
% w - (angular velocity of horizantal propellers)^2
% C - (angular velocit of vertical propellers)^2
%%%%%%%%%%%%%%%%%%%

ities in rad/s of the AUV propellers.
kf = 0.0019; % Motor Force Coeffecient
L = 0.4;    % Distance to propellers from center of gravity of AUV
A = [1 1; 1 -1]^-1;  % Inverse Force/Moment mapping matrix
B = [Fx/kf; Tr/(L*kf)]; % Desired Force matrix
w = A*B;    % Calculates the squared speeds of the two horizantal thrusters
C = Fz/(4*kf);  % Calculates the squared speeds of the four vertical thrusters

== matlab function UUV_PID_Control_Model/Global Transform ==
  data: u input; xdot output; psi input; ydot output
function [xdot,ydot] = fcn(u,psi)
%%%%%%%%%%%%%%%%%%%
% This function takes in the surge and psi orientation of the UUV and
% transforms it into the global velocities in the x and y direction
%%%%%%%%%%%%%%%%%%%
% Inputs: 
    % u - surge velocity of UUV
    % psi - orinetation of UUV about the z axis
%%%%%%%%%%%%%%%%%%%
% Outputs
    % xdot - global velocity in x direction
    % ydot - global velocity in y direction
%%%%%%%%%%%%%%%%%%

% Transformation
xdot=u*cos(psi);
ydot = u*sin(psi);

== matlab function UUV_PID_Control_Model/LOS guidance/alpha,e ==
  settings: updateMethod=DISCRETE
  data: x input; alpha output; y input; wp input; e output; r input; zd output; q output; eq output
function [alpha,e,zd,q,eq] = fcn(x,y,wp,r)
% fcn.m     e.anderlini@ucl.ac.uk      06/10/2017
%%%%%%%%%%%%%%%%%%%%%%%%%%%%%%%%%%%%%%%%%%%%%%%%%%%%%%%%%%%%%%%%%%%%%%%%%%%
% This function returns the angle alpha and the cross-track error.
% Input:
% x:  x-position;
% y:  y-position;
% wp: waypoints;
% r:  radius of acceptance.
%%%%%%%%%%%%%%%%%%%%%%%%%%%%%%%%%%%%%%%%%%%%%%%%%%%%%%%%%%%%%%%%%%%%%%%%%%%

%persistent k n alp;
% Initialize persistent variables:
%if isempty(k)
    %k = 1;
    %n = size(wp,1);
    alp = atan2(wp(2,2)-wp(1,2),wp(2,1)-wp(1,1));
%end

%{
% Check if k has to be updated:

    if ((wp(k+1,1)-x)^2+(wp(k+1,2)-y)^2) <= r^2
        k = k + 1;
        alp = atan2(wp(k+1,2)-wp(k,2),wp(k+1,1)-wp(k,1));
    end
end
%}

% Compute the cross-track error:
e = [-sin(alp),cos(alp)]*[wp(2,1)-x;wp(2,2)-y];
% Output the angle and desired depth as well:
alpha = alp;
zd = wp(2,3);

% Code for stopping sim
if sqrt((wp(2,1)-x)^2+(wp(2,2)-y)^2) <= r
    q = 0;
else 
    q=1;
end
eq = sqrt((wp(2,1)-x)^2+(wp(2,2)-y)^2)
